simulink model "sx2"  (R2015b)
settings: Solver=VariableStepAuto  StartTime=0.0  StopTime=0.01  RelTol=1e-3
settings Model: Creator=hohotulca  LastModifiedBy=hohotulca

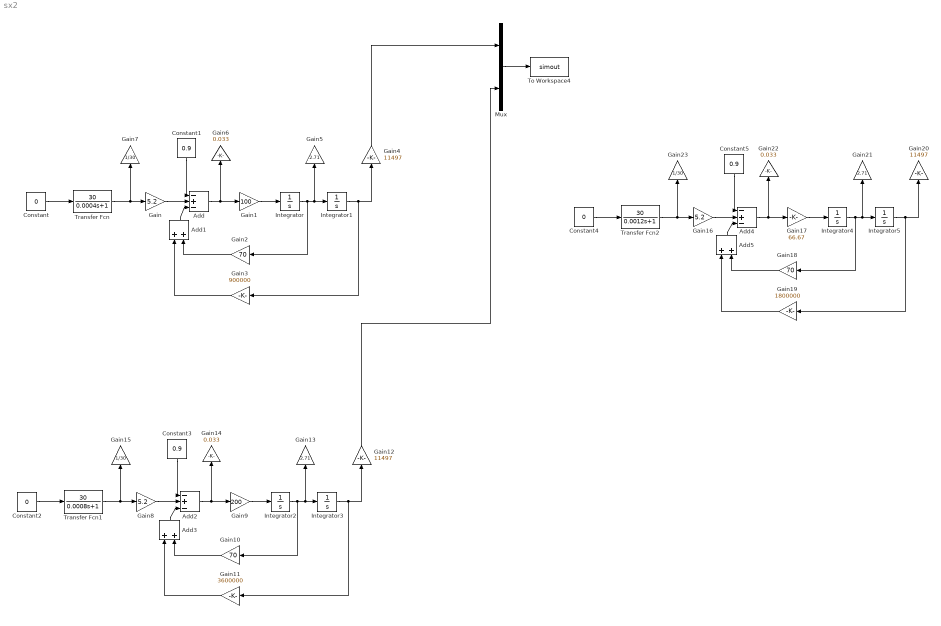
== system sx2 ==
  Add : Sum  Inputs=-+-
  Add1 : Sum
  Add2 : Sum  Inputs=-+-
  Add3 : Sum
  Add4 : Sum  Inputs=-+-
  Add5 : Sum
  Constant : Constant  Value=0
  Constant1 : Constant  Value=0.9
  Constant2 : Constant  Value=0
  Constant3 : Constant  Value=0.9
  Constant4 : Constant  Value=0
  Constant5 : Constant  Value=0.9
  Gain : Gain  Gain=5.2
  Gain1 : Gain  Gain=100
  Gain10 : Gain  Gain=70
  Gain11 : Gain  Gain=3600000
  Gain12 : Gain  Gain=11497
  Gain13 : Gain  Gain=2.71
  Gain14 : Gain  Gain=0.033
  Gain15 : Gain  Gain=1/30
  Gain16 : Gain  Gain=5.2
  Gain17 : Gain  Gain=66.67
  Gain18 : Gain  Gain=70
  Gain19 : Gain  Gain=1800000
  Gain2 : Gain  Gain=70
  Gain20 : Gain  Gain=11497
  Gain21 : Gain  Gain=2.71
  Gain22 : Gain  Gain=0.033
  Gain23 : Gain  Gain=1/30
  Gain3 : Gain  Gain=900000
  Gain4 : Gain  Gain=11497
  Gain5 : Gain  Gain=2.71
  Gain6 : Gain  Gain=0.033
  Gain7 : Gain  Gain=1/30
  Gain8 : Gain  Gain=5.2
  Gain9 : Gain  Gain=200
  Integrator{,1..5} (6 alike) : Integrator
  Mux : Mux  Inputs=2
  To Workspace4 : ToWorkspace  VariableName=simout  SaveFormat=Timeseries  SampleTime=-1
  Transfer Fcn : TransferFcn  Numerator=[30]  Denominator=[0.0004 1]
  Transfer Fcn1 : TransferFcn  Numerator=[30]  Denominator=[0.0008 1]
  Transfer Fcn2 : TransferFcn  Numerator=[30]  Denominator=[0.0012 1]
  wires:
  Constant/1 -> Transfer Fcn/1
  Transfer Fcn/1 -> Gain/1, Gain7/1
  Gain/1 -> Add/2
  Add/1 -> Gain1/1, Gain6/1
  Gain1/1 -> Integrator/1
  Integrator/1 -> Gain5/1, Integrator1/1, Gain2/1
  Gain2/1 -> Add1/2
  Add1/1 -> Add/3
  Gain3/1 -> Add1/1
  Integrator1/1 -> Gain3/1, Gain4/1
  Constant1/1 -> Add/1
  Constant2/1 -> Transfer Fcn1/1
  Transfer Fcn1/1 -> Gain8/1, Gain15/1
  Gain8/1 -> Add2/2
  Add2/1 -> Gain9/1, Gain14/1
  Gain9/1 -> Integrator2/1
  Integrator2/1 -> Gain13/1, Integrator3/1, Gain10/1
  Gain10/1 -> Add3/2
  Add3/1 -> Add2/3
  Gain11/1 -> Add3/1
  Integrator3/1 -> Gain11/1, Gain12/1
  Constant3/1 -> Add2/1
  Constant4/1 -> Transfer Fcn2/1
  Transfer Fcn2/1 -> Gain16/1, Gain23/1
  Gain16/1 -> Add4/2
  Add4/1 -> Gain17/1, Gain22/1
  Gain17/1 -> Integrator4/1
  Integrator4/1 -> Gain21/1, Integrator5/1, Gain18/1
  Gain18/1 -> Add5/2
  Add5/1 -> Add4/3
  Gain19/1 -> Add5/1
  Integrator5/1 -> Gain19/1, Gain20/1
  Constant5/1 -> Add4/1
  Mux/1 -> To Workspace4/1
  Gain4/1 -> Mux/1
  Gain12/1 -> Mux/2
